simulink model "parteB_performance"  (R2022b)
settings: Solver=ode4  StartTime=0.0  StopTime=375  FixedStep=0.125  RelTol=1e-3
libraries: fuzblock x1
settings Model: Creator=andre  LastModifiedBy=maria
settings SolverCC: AlgebraicLoopSolver=TrustRegion
settings DebuggingCC: UnconnectedInputMsg=warning  UnconnectedOutputMsg=warning  UnconnectedLineMsg=warning  SFMachineParentedDataDiag=warning
settings ModelReferenceCC: EnableRefExpFcnMdlSchedulingChecks=on

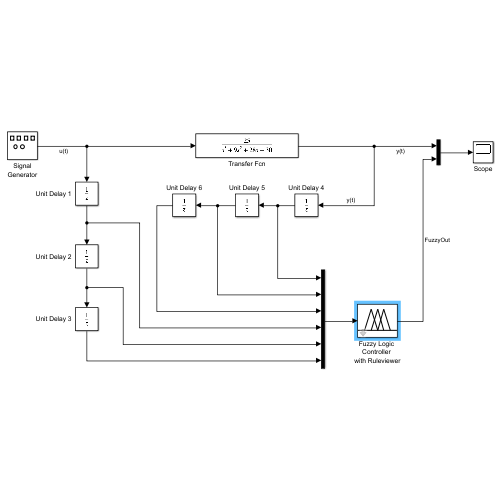
[thumbnail: Simulink's stored preview of the top-level diagram]
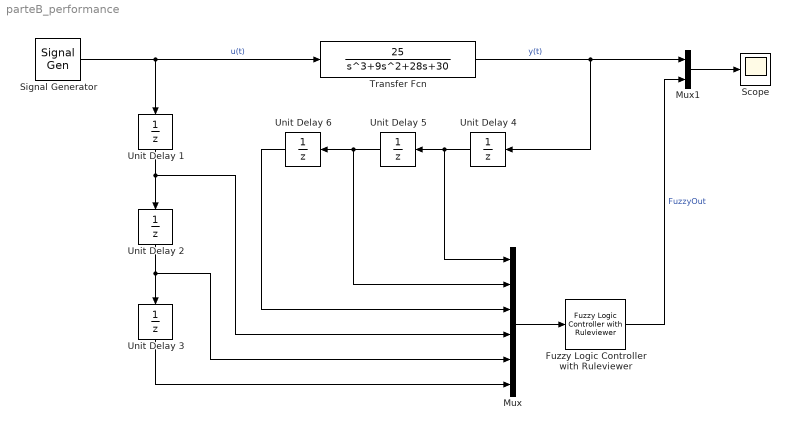
== system parteB_performance ==
  Fuzzy Logic Controller with Ruleviewer : fuzblock/Fuzzy Logic  Controller  with Ruleviewer  fismatrix=subB  Ts=1
  Mux : Mux  Inputs=6
  Mux1 : Mux  Inputs=2
  Scope : Scope
  Signal Generator : SignalGenerator  WaveForm=sawtooth  Frequency=0.05  Units=rad/sec
  Transfer Fcn : TransferFcn  Numerator=[25]  Denominator=[1 9 28 30]
  Unit Delay {1..6} (6 alike) : UnitDelay  SampleTime=0.125  HasFrameUpgradeWarning=on
  wires:
  Signal Generator/1 -> Unit Delay 1/1, Transfer Fcn/1  "u(t)"
  Transfer Fcn/1 -> Unit Delay 4/1, Mux1/1  "y(t)"
  Mux1/1 -> Scope/1
  Unit Delay 1/1 -> Unit Delay 2/1, Mux/4
  Unit Delay 2/1 -> Unit Delay 3/1, Mux/5
  Unit Delay 3/1 -> Mux/6
  Mux/1 -> Fuzzy Logic Controller with Ruleviewer/1
  Fuzzy Logic Controller with Ruleviewer/1 -> Mux1/2  "FuzzyOut"
  Unit Delay 4/1 -> Unit Delay 5/1, Mux/1
  Unit Delay 5/1 -> Unit Delay 6/1, Mux/2
  Unit Delay 6/1 -> Mux/3
